simulink model "gimbaledRocket3DOF"  (R2025b)
settings: Solver=VariableStepAuto  StartTime=0.0  StopTime=30  RelTol=1e-6
libraries: dspsrcs4 x1
settings Model: Creator=ghowa  LastModifiedBy=Gurjinder

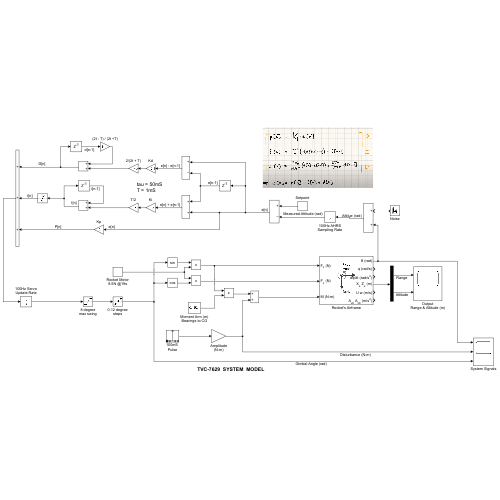
[thumbnail: Simulink's stored preview of the top-level diagram]
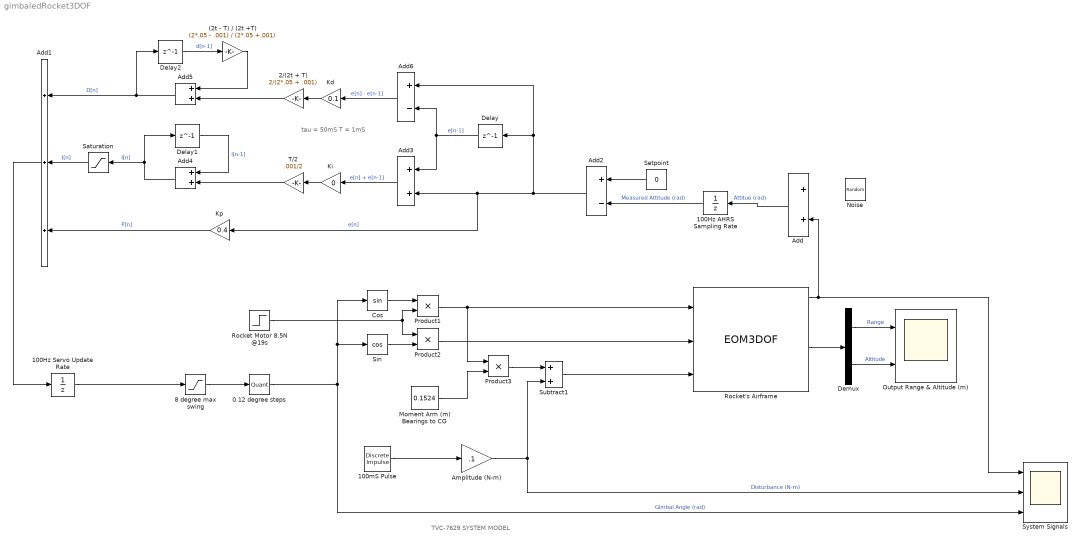
== system gimbaledRocket3DOF ==
  note: tau = 50mS
      | T = 1mS
  note: TVC-7629 SYSTEM MODEL
  (2t - T) / (2t +T) : Gain  Gain=(2*.05 - .001) / (2*.05 +.001)
  0.12 degree steps : Quantizer  QuantizationInterval=0.0021
  100Hz AHRS Sampling Rate : UnitDelay  SampleTime=.01  HasFrameUpgradeWarning=on
  100Hz Servo Update Rate : UnitDelay  SampleTime=.01  HasFrameUpgradeWarning=on
  100mS Pulse : dspsrcs4/Discrete  Impulse  SFcnStateName=COUNT  Delay=10  SampleTime=.1  FrameSample=1  OutputFrames=off  dataType=double  isSigned=on  wordLen=16  udDataType=sfix(16)  fracBitsMode=Best precision  numFracBits=15  OutDataTypeStr=double  LastOutDataTypeStr=double
      settings: SFcnIsStateOwnerBlock=on
  2/(2t + T) : Gain  Gain=2/(2*.05 + .001)
  8 degree max swing : Saturate  UpperLimit=0.14  LowerLimit=-0.14
  Add{,3..5} (4 alike) : Sum
  Add1 : Sum  Inputs=+++
  Add2 : Sum  Inputs=+-
  Add6 : Sum  Inputs=+-
  Amplitude (N-m) : Gain  Gain=.1
  Cos : Trigonometry
  Delay : Delay  DelayLength=1  InitialCondition=0  SampleTime=.001
  Delay1 : Delay  DelayLength=1  InitialCondition=0  SampleTime=.001
  Delay2 : Delay  DelayLength=1  InitialCondition=0  SampleTime=.001
  Demux : Demux  Outputs=2
  Kd : Gain  Gain=0.1
  Ki : Gain  Gain=0
  Kp : Gain  Gain=0.4
  Moment Arm (m) Bearings to CG : Constant  Value=0.1524
  Noise : UniformRandomNumber  Minimum=-0.0017  Maximum=0.0017  SampleTime=0.001
  Output Range & Altitude (m) : Scope  NumInputPorts=2
      settings: ActiveDisplayYMinimum=-36.910267667686753  ActiveDisplayYMaximum=293.15029678358394
  Product1 : Product
  Product2 : Product
  Product3 : Product
  Rocket Motor 8.5N @19s : Step  Time=19  Before=8.5  After=0  SampleTime=0
  Rocket's Airframe : EOM3DOF  v_ini=0  mass=0.771  Iyy=0.0126  g=-9.81
  Saturation : Saturate  UpperLimit=3  LowerLimit=-3
  Setpoint : Constant  Value=0
  Sin : Trigonometry  Operator=cos
  Subtract1 : Sum
  System Signals : Scope  NumInputPorts=3
      settings: ActiveDisplayYMinimum=-0.0665560507610336  ActiveDisplayYMaximum=0.090334101245009263
  T/2 : Gain  Gain=.001/2
  wires:
  Rocket Motor 8.5N @19s/1 -> Product2/1, Product1/2
  Demux/1 -> Output Range & Altitude (m)/1  "Range"
  Demux/2 -> Output Range & Altitude (m)/2  "Altitude"
  100Hz AHRS Sampling Rate/1 -> Add2/2  "Measured Attitude (rad)"
  100mS Pulse/1 -> Amplitude (N-m)/1
  8 degree max swing/1 -> 0.12 degree steps/1
  0.12 degree steps/1 -> Cos/1, Sin/1, System Signals/3  "Gimbal Angle (rad)"
  Amplitude (N-m)/1 -> Subtract1/2, System Signals/2  "Disturbance (N-m)"
  Cos/1 -> Product1/1
  Sin/1 -> Product2/2
  Product1/1 -> Rocket's Airframe/1, Product3/1
  Product3/1 -> Subtract1/1
  Moment Arm (m) Bearings to CG/1 -> Product3/2
  Subtract1/1 -> Rocket's Airframe/3
  Product2/1 -> Rocket's Airframe/2
  Rocket's Airframe/4 -> Demux/1
  Add/1 -> 100Hz AHRS Sampling Rate/1  "Attitue (rad)"
  Add5/1 -> Add1/1, Delay2/1  "D[n]"
  Add4/1 -> Saturation/1, Delay1/1  "I[n]"
  Setpoint/1 -> Add2/1
  Delay2/1 -> (2t - T) / (2t +T)/1  "d[n-1]"
  Kd/1 -> 2/(2t + T)/1
  Delay/1 -> Add3/1, Add6/2  "e[n-1]"
  Add2/1 -> Add3/2, Kp/1, Delay/1, Add6/1  "e[n]"
  Ki/1 -> T/2/1
  Add3/1 -> Ki/1  "e[n] + e[n-1]"
  2/(2t + T)/1 -> Add5/2
  (2t - T) / (2t +T)/1 -> Add5/1
  T/2/1 -> Add4/2
  Delay1/1 -> Add4/1  "i[n-1]"
  Kp/1 -> Add1/3  "P[n]"
  Saturation/1 -> Add1/2  "I[n]"
  Add6/1 -> Kd/1  "e[n] - e[n-1]"
  Add1/1 -> 100Hz Servo Update Rate/1
  100Hz Servo Update Rate/1 -> 8 degree max swing/1
  Rocket's Airframe/1 -> Add/2, System Signals/1
